simulink model "nonlinear_model_pin"  (R2025a)
settings: Solver=VariableStepAuto  StartTime=0.0  StopTime=10.0  RelTol=1e-3
settings Model: Creator=khanh  LastModifiedBy=khanh

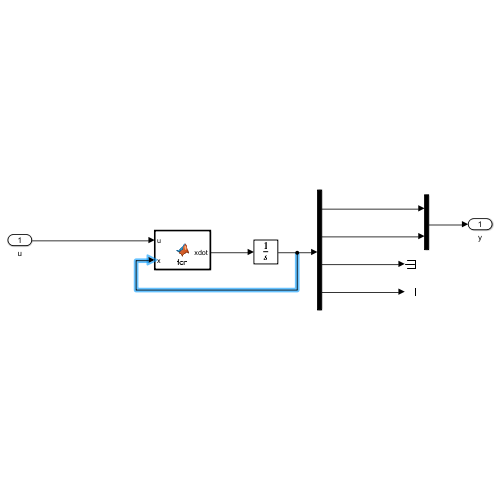
[thumbnail: Simulink's stored preview of the top-level diagram]
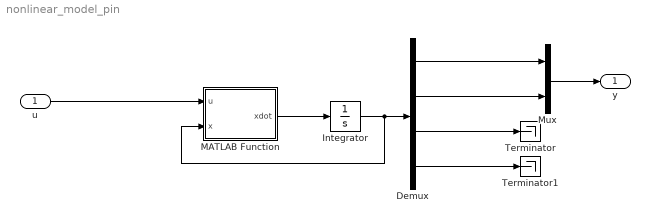
== system nonlinear_model_pin ==
  u : Inport  PortDimensions=2
  Demux : Demux
  Integrator : Integrator  InitialCondition=zeros(4,1)
  MATLAB Function : MATLAB Function  TreatAsAtomicUnit=on
  Mux : Mux  Inputs=2
  Terminator : Terminator
  Terminator1 : Terminator
  y : Outport
  wires:
  u/1 -> MATLAB Function/1(u)
  MATLAB Function/1(xdot) -> Integrator/1
  Integrator/1 -> MATLAB Function/2(x), Demux/1
  Demux/3 -> Terminator/1
  Demux/4 -> Terminator1/1
  Demux/1 -> Mux/1
  Demux/2 -> Mux/2
  Mux/1 -> y/1

== matlab function nonlinear_model_pin/MATLAB Function ==
  data: u input size=2; xdot output size=4; x input size=4
function xdot  = fcn(u, x)

theta = x(1);
psi = x(2);
theta_dot = x(3);
psi_dot = x(4);

Vp = u(1);
Vy = u(2);

% Parameters
% distance from pivot to center of rotor/propeller (m)
Dt = 0.16743; 
% total aero body mass (kg)
Mb = 1.07; 
% distance from aero body plane to center of mass below (m)
l = 2.4e-3; 
% Moment of inertia about pitch-axis (kg-m^2)
Jp = 23188500.45 / 1000 * 0.001^2; % from CAD: 23188500.45 g-mm^2
% Moment of inertia about pitch-axis (kg-m^2)
Jy = 23810415.95 / 1000 * 0.001^2; % from CAD: 23810415.95 g-mm^2;
% Gravity (m/s^2)
g = 9.81;
% Stiffness (N-m/V)
Ksp = 0.00744;
% Damping (N-m/V)
Dp = 0.00199;
% Pitch thrust gain (N/V)
Kpp = 0.00321;
% Pitch from yaw thrust gain (N/V)
Kpy = 0.00137;
% Damping (N-m/V)
Dy = 0.00192;
% Thrust (N-m/V)
Kyy = 0.00610;
% Yaw from pitch thrust gain (N/V)
Kyp = -0.00319;

theta_ddot = (Dt*Kpp*Vp + ...
              Dt*Kpy*Vy - ...
              Mb*g*l*cos(theta) - ...
              Dp*theta_dot - ...
              Ksp*theta - ...
              Mb*psi_dot^2*l^2*sin(theta)*cos(theta)) / (Jp + Mb*l^2);
psi_ddot = (Dt*Kyp*Vp + ...
            Kyy*Vy - ...
            Dy*psi_dot + ...
            Mb*l^2*psi_dot*theta_dot*sin(2*theta)) / (Jy + Mb*l^2*cos(theta)^2);

xdot = [theta_dot, psi_dot, theta_ddot, psi_ddot]';
